simulink model "wind_draiden_proto"  (R2020a)
settings: Solver=ode45  StartTime=0.0  StopTime=20  MaxStep=0.1  RelTol=1e-2  EnableMultiTasking=on
undefined symbols (not defined in the file or in its folder): ln
libraries: simulink x16
settings Model: Creator=Andrey  LastModifiedBy=Tamer
settings SolverCC: AlgebraicLoopSolver=LineSearch
settings DataIOCC: LimitDataPoints=on  SaveFormat=Array  SignalLoggingSaveFormat=ModelDataLogs  ReturnWorkspaceOutputs=off
settings OptimizationCC: InitFltsAndDblsToZero=on  EfficientMapNaN2IntZero=off  LifeSpan=inf
settings DebuggingCC: SaveWithParameterizedLinksMsg=none  UnderspecifiedInitializationDetection=Classic  MergeDetectMultiDrivingBlocksExec=none  SignalResolutionControl=TryResolveAllWithWarning  MaxConsecutiveZCsMsg=none  SolverPrmCheckMsg=warning  MultiTaskDSMMsg=warning  MultiTaskCondExecSysMsg=none  FcnCallInpInsideContextMsg=warning  StateNameClashWarn=warning  SFUnexpectedBacktrackingDiag=warning  SFNoUnconditionalDefaultTransitionDiag=warning  SFExecutionAtInitializationDiag=none  ArithmeticOperatorsInVariantConditions=warning
settings HardwareCC: ProdBitPerPointer=32  ProdBitPerSizeT=32  ProdBitPerPtrDiffT=32  ProdLargestAtomicFloat=None  ProdIntDivRoundTo=Undefined  ProdEndianess=Unspecified  ProdWordSize=32  ProdHWDeviceType=32-bit Generic  TargetBitPerPointer=64  TargetBitPerSizeT=64  TargetBitPerPtrDiffT=64  TargetLongLongMode=on  TargetIntDivRoundTo=Zero  TargetEndianess=LittleEndian  TargetWordSize=64  TargetHWDeviceType=MATLAB Host  ProdEqTarget=off
settings ModelReferenceCC: PropagateSignalLabelsOutOfModel=off
settings SFSimCC: SimUseLocalCustomCode=off  CustomCodeUndefinedFunction=UseInterfaceOnly
settings RTWCC: RTWUseLocalCustomCode=off
settings CodeAppCC: MaxIdLength=128
settings GRTTargetCC: TargetLangStandard=C89/C90 (ANSI)  CombineOutputUpdateFcns=off  GRTInterface=on
settings ConfigComp: CovMetricSettings=dw  CovHtmlReporting=on  CovSaveCumulativeToWorkspaceVar=on  CovSaveSingleToWorkspaceVar=on  CovExternalEMLEnable=off

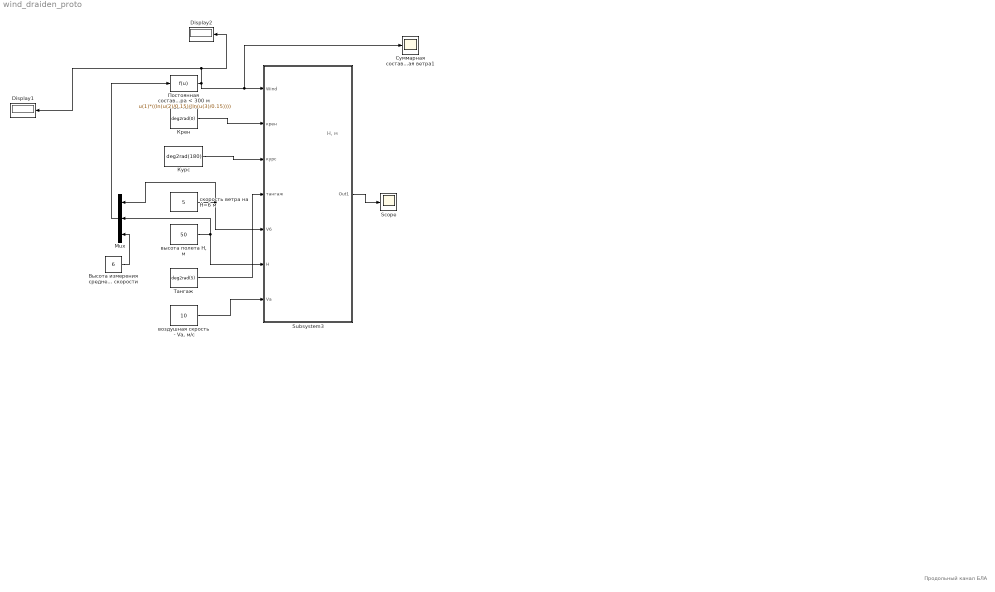
== system wind_draiden_proto ==
  note: Н, м
  note: Продольный канал БЛА
  "    Постоянная составляющая скорости ветра < 300 м" : Fcn  Expr=u(1)*((ln(u(2)/0.15)/(ln(u(3)/0.15))))
  Display1 : Display
  Display2 : Display
  Mux : Mux  Inputs=3
  Scope : Scope
  Subsystem3 : Subsystem
  Высота измерения среднегодовой скорости : Constant  Value=6
  "Крен " : Constant  Value=deg2rad(0)
  Курс : Constant  Value=deg2rad(180)
  Суммарная составляющая ветра1 : Scope
  Тангаж : Constant  Value=deg2rad(5)
  "воздушная скрость  - Vа, м/с" : Constant  Value=10
  "высота полета Н, м " : Constant  Value=50
  "скорость ветра на Н=6 м " : Constant  Value=5
  wires:
  Subsystem3/1(Out1) -> Scope/1
  "Крен "/1 -> Subsystem3/2(крен)
  Курс/1 -> Subsystem3/3(курс)
  "скорость ветра на Н=6 м "/1 -> Subsystem3/5(V6), Mux/1
  "высота полета Н, м "/1 -> Subsystem3/6(H), Mux/2
  Тангаж/1 -> Subsystem3/4("тангаж ")
  "    Постоянная составляющая скорости ветра < 300 м"/1 -> Display2/1, Display1/1, Суммарная составляющая ветра1/1, Subsystem3/1(Wind)
  Высота измерения среднегодовой скорости/1 -> Mux/3
  Mux/1 -> "    Постоянная составляющая скорости ветра < 300 м"/1
  "воздушная скрость  - Vа, м/с"/1 -> Subsystem3/7(Va)

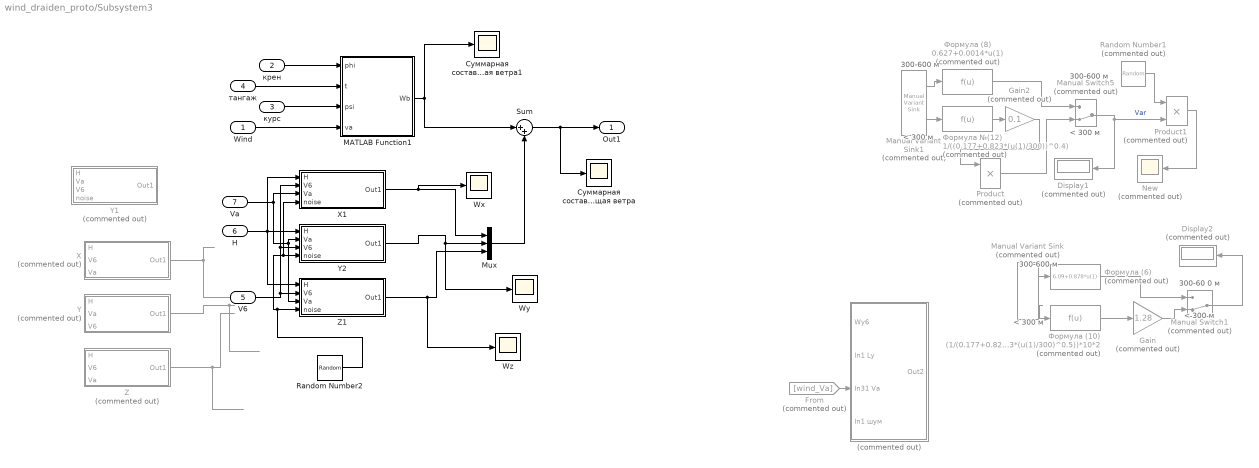
== system wind_draiden_proto/Subsystem3 ==
  note: < 300 м
  note: < 300 м
  note: 300-600 м
  note: < 300 м
  note: 300-60 0 м
  note: 300-600 м
  note: < 300 м
  note: 300-600 м
  Wind : Inport
  крен : Inport  Port=2
  курс : Inport  Port=3
  "тангаж " : Inport  Port=4
  V6 : Inport  Port=5
  H : Inport  Port=6
  Va : Inport  Port=7
  " " : Subsystem  Commented=on
  Display1 : Display  Commented=on
  Display2 : Display  Commented=on
  From : From  Commented=on  GotoTag=wind_Va
  Gain : Gain  Commented=on  Gain=1.28
  Gain2 : Gain  Commented=on  Gain=0.1
  MATLAB Function1 : MATLAB Function  TreatAsAtomicUnit=on
  Manual Variant Sink : simulink/Signal Routing/Manual Variant Sink  Commented=on  NumChoices=2  LabelModeActiveChoice=V_2
  Manual Variant Sink1 : simulink/Signal Routing/Manual Variant Sink  Commented=on  NumChoices=2  LabelModeActiveChoice=V_2
  Manual Switch1 : ManualSwitch  Commented=on  CurrentSetting=0
  Manual Switch5 : ManualSwitch  Commented=on  CurrentSetting=0
  Mux : Mux  Inputs=3
  New : Scope  Commented=on
  Product : Product  Commented=on
  Product1 : Product  Commented=on
  Random Number1 : RandomNumber  Commented=on  SampleTime=0.1
  Random Number2 : RandomNumber  SampleTime=0.1
  Sum : Sum  Inputs=|++
  Wx : Scope
  Wy : Scope
  Wz : Scope
  X : Subsystem  Commented=on  TreatAsAtomicUnit=on
  X1 : Subsystem  TreatAsAtomicUnit=on
  Y : Subsystem  Commented=on  TreatAsAtomicUnit=on
  Y1 : Subsystem  Commented=on  TreatAsAtomicUnit=on
  Y2 : Subsystem  TreatAsAtomicUnit=on
  Z : Subsystem  Commented=on  TreatAsAtomicUnit=on
  Z1 : Subsystem  TreatAsAtomicUnit=on
  Суммарная составляющая ветра : Scope
  Суммарная составляющая ветра1 : Scope
  Формула (10) : Fcn  Commented=on  Expr=(1/(0.177+0.823*(u(1)/300)^0.5))*10*2
  Формула (6) : Fcn  Commented=on  Expr=6.09+0.878*u(1)
  Формула (8) : Fcn  Commented=on  Expr=0.627+0.0014*u(1)
  Формула №(12) : Fcn  Commented=on  Expr=1/((0.177+0.823*(u(1)/300))^0.4)
  Out1 : Outport
  wires:
  Формула (10)/1 -> Gain/1
  Manual Variant Sink/1 -> Формула (6)/1
  Manual Variant Sink/2 -> Формула (10)/1
  крен/1 -> MATLAB Function1/1(phi)
  курс/1 -> MATLAB Function1/3(psi)
  Wind/1 -> MATLAB Function1/4(va)
  Gain2/1 -> Product/1
  Manual Variant Sink1/1 -> Формула (8)/1
  Формула (8)/1 -> Manual Switch5/1
  Формула №(12)/1 -> Gain2/1
  Product/1 -> Manual Switch5/2
  Manual Variant Sink1/2 -> Формула №(12)/1
  Manual Switch5/1 -> Product1/2, Display1/1  "Var"
  Формула (6)/1 -> Manual Switch1/1
  Gain/1 -> Manual Switch1/2
  "тангаж "/1 -> MATLAB Function1/2(t)
  From/1 -> " "/3(In31 Va)
  Manual Switch1/1 -> Display2/1
  Product1/1 -> New/1
  Random Number1/1 -> Product1/1
  MATLAB Function1/1(Wb) -> Sum/1, Суммарная составляющая ветра1/1
  Mux/1 -> Sum/2
  Sum/1 -> Суммарная составляющая ветра/1, Out1/1
  Z/1(Out1) -> ?
  X/1(Out1) -> ?
  Y/1(Out1) -> ?
  Va/1 -> Y2/2(Va), Z1/3(Va), X1/3(Va)
  H/1 -> Y2/1(H), X1/1(H), Z1/1(H)
  V6/1 -> X1/2(V6), Y2/3(V6), Z1/2(V6)
  Z1/1(Out1) -> Wz/1, Mux/3
  X1/1(Out1) -> Mux/1, Wx/1
  Y2/1(Out1) -> Mux/2, Wy/1
  Random Number2/1 -> Y2/4(noise), X1/4(noise), Z1/4(noise)

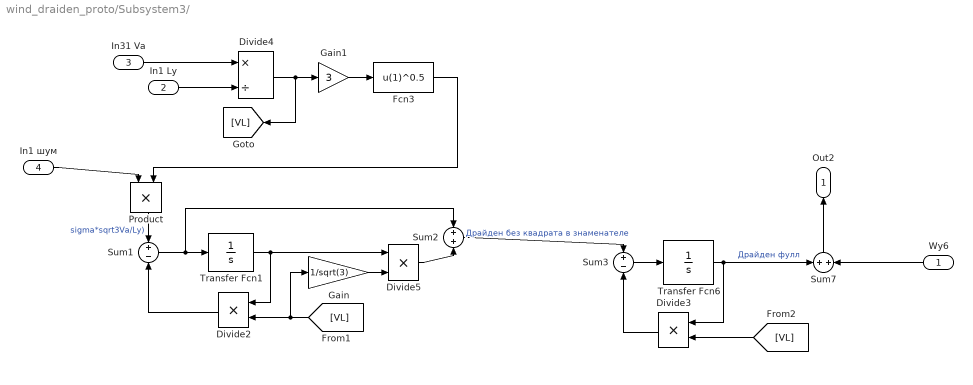
== system wind_draiden_proto/Subsystem3/  ==
  Wy6 : Inport
  In1 Ly : Inport  Port=2
  In31 Va : Inport  Port=3
  "In1 шум " : Inport  Port=4
  Divide2 : Product  Inputs=**
  Divide3 : Product  Inputs=**
  Divide4 : Product  Inputs=*/
  Divide5 : Product  Inputs=**
  Fcn3 : Fcn  Expr=u(1)^0.5
  Gain : Gain  Gain=1/sqrt(3)
  Gain1 : Gain  Gain=3
  Product : Product
  Sum1 : Sum  Inputs=+-
  Sum2 : Sum
  Sum3 : Sum  Inputs=+-
  Sum7 : Sum
  Transfer Fcn1 : TransferFcn  Denominator="[1  0]"
  Transfer Fcn6 : TransferFcn  Denominator="[1  0]"
  Out2 : Outport
  wires:
  Divide4/1 -> [VL], Gain1/1
  Sum1/1 -> Transfer Fcn1/1, Sum2/1
  Sum2/1 -> Sum3/1  "Драйден без квадрата в знаменателе"
  Transfer Fcn1/1 -> Divide2/1, Divide5/1
  Divide2/1 -> Sum1/2
  Gain1/1 -> Fcn3/1
  In31 Va/1 -> Divide4/1
  In1 Ly/1 -> Divide4/2
  [VL] -> Gain/1, Divide2/2
  Gain/1 -> Divide5/2
  Divide5/1 -> Sum2/2
  Transfer Fcn6/1 -> Sum7/1, Divide3/1  "Драйден фулл"
  Divide3/1 -> Sum3/2
  Sum3/1 -> Transfer Fcn6/1
  [VL] -> Divide3/2
  Wy6/1 -> Sum7/2
  Sum7/1 -> Out2/1
  "In1 шум "/1 -> Product/1
  Fcn3/1 -> Product/2
  Product/1 -> Sum1/1  "sigma*sqrt3Va/Ly)"

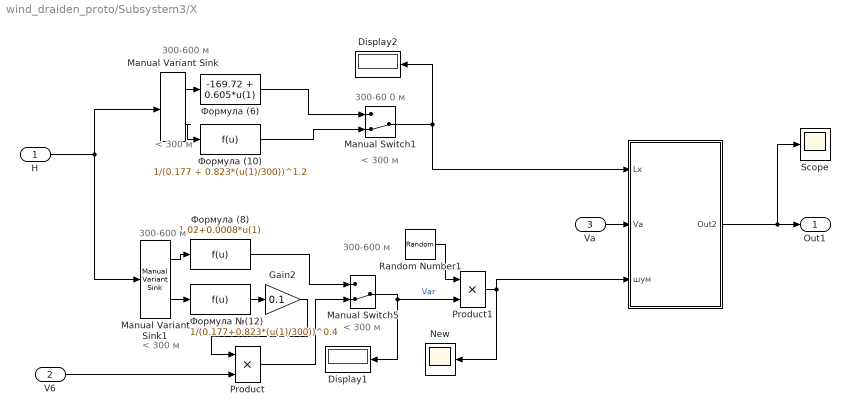
== system wind_draiden_proto/Subsystem3/X ==
  note: < 300 м
  note: 300-600 м
  note: < 300 м
  note: < 300 м
  note: 300-600 м
  note: < 300 м
  note: 300-60 0 м
  note: 300-600 м
  H : Inport
  V6 : Inport  Port=2
  Va : Inport  Port=3
  " " : Subsystem
  Display1 : Display
  Display2 : Display
  Gain2 : Gain  Gain=0.1
  Manual Variant Sink : simulink/Signal Routing/Manual Variant Sink  NumChoices=2  LabelModeActiveChoice=V_2
  Manual Variant Sink1 : simulink/Signal Routing/Manual Variant Sink  NumChoices=2  LabelModeActiveChoice=V_2
  Manual Switch1 : ManualSwitch  CurrentSetting=0
  Manual Switch5 : ManualSwitch  CurrentSetting=0
  New : Scope
  Product : Product
  Product1 : Product
  Random Number1 : RandomNumber  SampleTime=0.1
  Scope : Scope
  Формула (10) : Fcn  Expr=1/(0.177 + 0.823*(u(1)/300))^1.2
  Формула (6) : Fcn  Expr=-169.72 + 0.605*u(1)
  Формула (8) : Fcn  Expr=1.02+0.0008*u(1)
  Формула №(12) : Fcn  Expr=1/(0.177+0.823*(u(1)/300))^0.4
  Out1 : Outport
  wires:
  Random Number1/1 -> Product1/1
  Формула №(12)/1 -> Gain2/1
  Формула (8)/1 -> Manual Switch5/1
  Product1/1 -> New/1, " "/3("шум ")
  Manual Variant Sink/2 -> Формула (10)/1
  Manual Variant Sink1/1 -> Формула (8)/1
  Gain2/1 -> Product/1
  Manual Variant Sink1/2 -> Формула №(12)/1
  Manual Switch5/1 -> Product1/2, Display1/1  "Var"
  " "/1(Out2) -> Scope/1, Out1/1
  Product/1 -> Manual Switch5/2
  Формула (6)/1 -> Manual Switch1/1
  H/1 -> Manual Variant Sink1/1, Manual Variant Sink/1
  V6/1 -> Product/2
  Manual Variant Sink/1 -> Формула (6)/1
  Manual Switch1/1 -> " "/1(Lx), Display2/1
  Формула (10)/1 -> Manual Switch1/2
  Va/1 -> " "/2(Va)

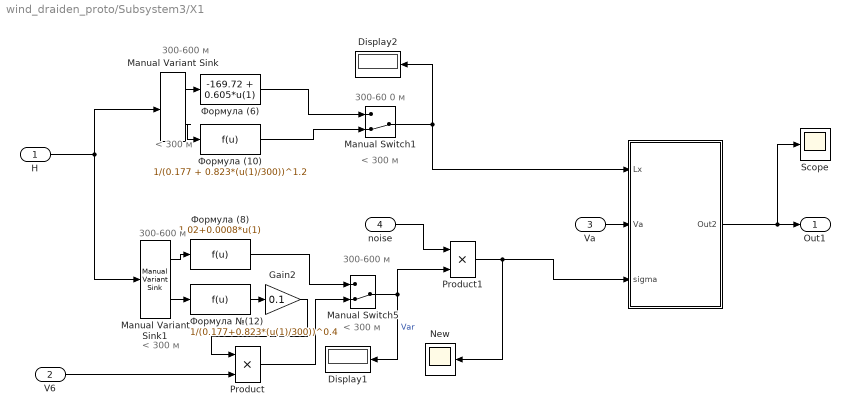
== system wind_draiden_proto/Subsystem3/X1 ==
  note: < 300 м
  note: 300-600 м
  note: < 300 м
  note: < 300 м
  note: 300-600 м
  note: < 300 м
  note: 300-60 0 м
  note: 300-600 м
  H : Inport
  V6 : Inport  Port=2
  Va : Inport  Port=3
  noise : Inport  Port=4
  " " : Subsystem
  Display1 : Display
  Display2 : Display
  Gain2 : Gain  Gain=0.1
  Manual Variant Sink : simulink/Signal Routing/Manual Variant Sink  NumChoices=2  LabelModeActiveChoice=V_2
  Manual Variant Sink1 : simulink/Signal Routing/Manual Variant Sink  NumChoices=2  LabelModeActiveChoice=V_2
  Manual Switch1 : ManualSwitch  CurrentSetting=0
  Manual Switch5 : ManualSwitch  CurrentSetting=0
  New : Scope
  Product : Product
  Product1 : Product
  Scope : Scope
  Формула (10) : Fcn  Expr=1/(0.177 + 0.823*(u(1)/300))^1.2
  Формула (6) : Fcn  Expr=-169.72 + 0.605*u(1)
  Формула (8) : Fcn  Expr=1.02+0.0008*u(1)
  Формула №(12) : Fcn  Expr=1/(0.177+0.823*(u(1)/300))^0.4
  Out1 : Outport
  wires:
  Формула №(12)/1 -> Gain2/1
  Формула (8)/1 -> Manual Switch5/1
  Manual Variant Sink/2 -> Формула (10)/1
  Manual Variant Sink1/1 -> Формула (8)/1
  Gain2/1 -> Product/1
  Manual Variant Sink1/2 -> Формула №(12)/1
  Manual Switch5/1 -> Display1/1, Product1/2  "Var"
  " "/1(Out2) -> Scope/1, Out1/1
  Product/1 -> Manual Switch5/2
  Формула (6)/1 -> Manual Switch1/1
  H/1 -> Manual Variant Sink1/1, Manual Variant Sink/1
  V6/1 -> Product/2
  Manual Variant Sink/1 -> Формула (6)/1
  Manual Switch1/1 -> " "/1(Lx), Display2/1
  Формула (10)/1 -> Manual Switch1/2
  Va/1 -> " "/2(Va)
  Product1/1 -> New/1, " "/3("sigma ")
  noise/1 -> Product1/1

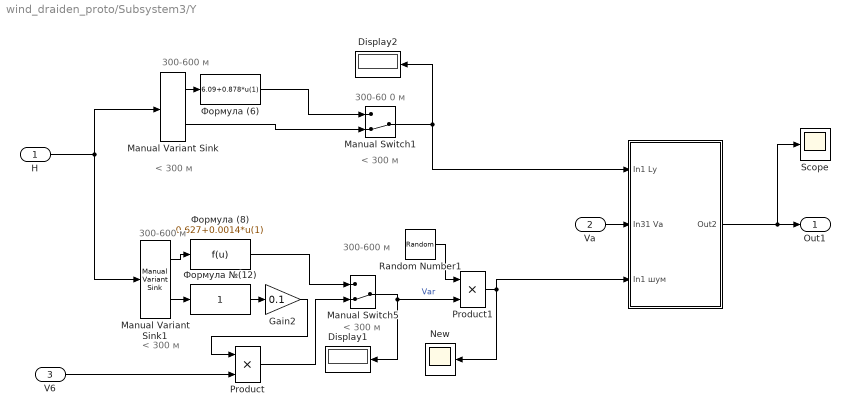
== system wind_draiden_proto/Subsystem3/Y ==
  note: < 300 м
  note: 300-600 м
  note: < 300 м
  note: < 300 м
  note: 300-600 м
  note: < 300 м
  note: 300-60 0 м
  note: 300-600 м
  H : Inport
  Va : Inport  Port=2
  V6 : Inport  Port=3
  " " : Subsystem
  Display1 : Display
  Display2 : Display
  Gain2 : Gain  Gain=0.1
  Manual Variant Sink : simulink/Signal Routing/Manual Variant Sink  NumChoices=2  LabelModeActiveChoice=V_2
  Manual Variant Sink1 : simulink/Signal Routing/Manual Variant Sink  NumChoices=2  LabelModeActiveChoice=V_2
  Manual Switch1 : ManualSwitch  CurrentSetting=0
  Manual Switch5 : ManualSwitch  CurrentSetting=0
  New : Scope
  Product : Product
  Product1 : Product
  Random Number1 : RandomNumber  SampleTime=0.1
  Scope : Scope
  Формула (6) : Fcn  Expr=6.09+0.878*u(1)
  Формула (8) : Fcn  Expr=0.627+0.0014*u(1)
  Формула №(12) : Fcn  Expr=1
  Out1 : Outport
  wires:
  Random Number1/1 -> Product1/1
  Формула №(12)/1 -> Gain2/1
  Формула (8)/1 -> Manual Switch5/1
  Product1/1 -> New/1, " "/3("In1 шум ")
  Manual Variant Sink1/1 -> Формула (8)/1
  Gain2/1 -> Product/1
  Manual Variant Sink1/2 -> Формула №(12)/1
  Manual Switch5/1 -> Product1/2, Display1/1  "Var"
  " "/1(Out2) -> Scope/1, Out1/1
  Product/1 -> Manual Switch5/2
  Формула (6)/1 -> Manual Switch1/1
  H/1 -> Manual Variant Sink1/1, Manual Variant Sink/1
  V6/1 -> Product/2
  Manual Variant Sink/1 -> Формула (6)/1
  Manual Switch1/1 -> " "/1(In1 Ly), Display2/1
  Manual Variant Sink/2 -> Manual Switch1/2
  Va/1 -> " "/2(In31 Va)

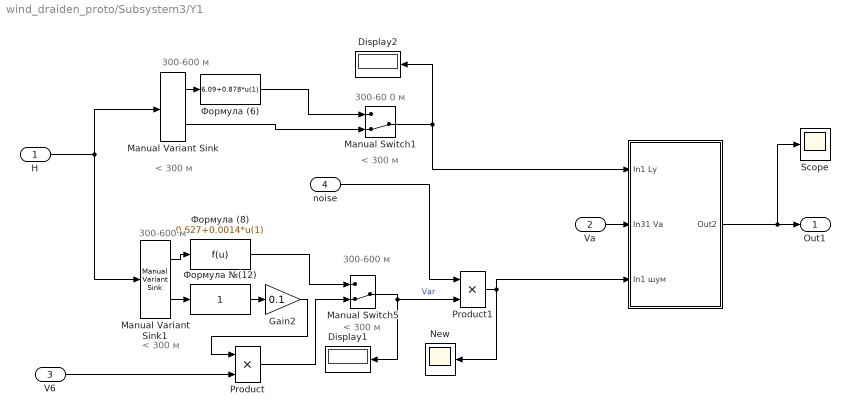
== system wind_draiden_proto/Subsystem3/Y1 ==
  note: < 300 м
  note: 300-600 м
  note: < 300 м
  note: < 300 м
  note: 300-600 м
  note: < 300 м
  note: 300-60 0 м
  note: 300-600 м
  H : Inport
  Va : Inport  Port=2
  V6 : Inport  Port=3
  noise : Inport  Port=4
  " " : Subsystem
  Display1 : Display
  Display2 : Display
  Gain2 : Gain  Gain=0.1
  Manual Variant Sink : simulink/Signal Routing/Manual Variant Sink  NumChoices=2  LabelModeActiveChoice=V_2
  Manual Variant Sink1 : simulink/Signal Routing/Manual Variant Sink  NumChoices=2  LabelModeActiveChoice=V_2
  Manual Switch1 : ManualSwitch  CurrentSetting=0
  Manual Switch5 : ManualSwitch  CurrentSetting=0
  New : Scope
  Product : Product
  Product1 : Product
  Scope : Scope
  Формула (6) : Fcn  Expr=6.09+0.878*u(1)
  Формула (8) : Fcn  Expr=0.627+0.0014*u(1)
  Формула №(12) : Fcn  Expr=1
  Out1 : Outport
  wires:
  noise/1 -> Product1/1
  Формула №(12)/1 -> Gain2/1
  Формула (8)/1 -> Manual Switch5/1
  Product1/1 -> " "/3("In1 шум "), New/1
  Manual Variant Sink1/1 -> Формула (8)/1
  Gain2/1 -> Product/1
  Manual Variant Sink1/2 -> Формула №(12)/1
  Manual Switch5/1 -> Product1/2, Display1/1  "Var"
  " "/1(Out2) -> Scope/1, Out1/1
  Product/1 -> Manual Switch5/2
  Формула (6)/1 -> Manual Switch1/1
  H/1 -> Manual Variant Sink1/1, Manual Variant Sink/1
  V6/1 -> Product/2
  Manual Variant Sink/1 -> Формула (6)/1
  Manual Switch1/1 -> " "/1(In1 Ly), Display2/1
  Manual Variant Sink/2 -> Manual Switch1/2
  Va/1 -> " "/2(In31 Va)

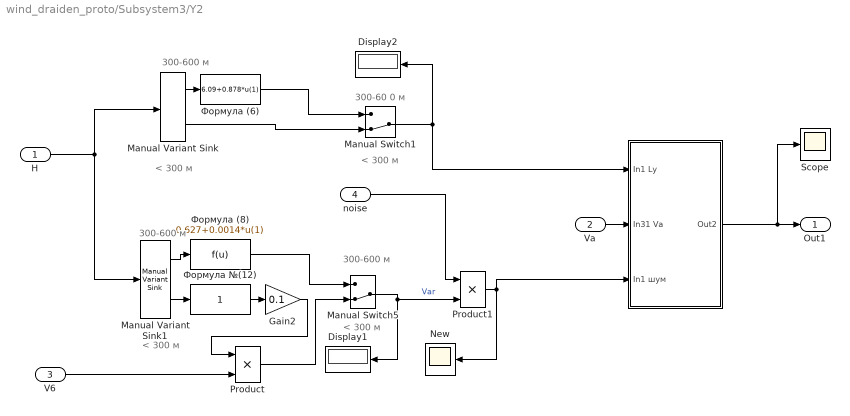
== system wind_draiden_proto/Subsystem3/Y2 ==
  note: < 300 м
  note: 300-600 м
  note: < 300 м
  note: < 300 м
  note: 300-600 м
  note: < 300 м
  note: 300-60 0 м
  note: 300-600 м
  H : Inport
  Va : Inport  Port=2
  V6 : Inport  Port=3
  noise : Inport  Port=4
  " " : Subsystem
  Display1 : Display
  Display2 : Display
  Gain2 : Gain  Gain=0.1
  Manual Variant Sink : simulink/Signal Routing/Manual Variant Sink  NumChoices=2  LabelModeActiveChoice=V_2
  Manual Variant Sink1 : simulink/Signal Routing/Manual Variant Sink  NumChoices=2  LabelModeActiveChoice=V_2
  Manual Switch1 : ManualSwitch  CurrentSetting=0
  Manual Switch5 : ManualSwitch  CurrentSetting=0
  New : Scope
  Product : Product
  Product1 : Product
  Scope : Scope
  Формула (6) : Fcn  Expr=6.09+0.878*u(1)
  Формула (8) : Fcn  Expr=0.627+0.0014*u(1)
  Формула №(12) : Fcn  Expr=1
  Out1 : Outport
  wires:
  noise/1 -> Product1/1
  Формула №(12)/1 -> Gain2/1
  Формула (8)/1 -> Manual Switch5/1
  Product1/1 -> New/1, " "/3("In1 шум ")
  Manual Variant Sink1/1 -> Формула (8)/1
  Gain2/1 -> Product/1
  Manual Variant Sink1/2 -> Формула №(12)/1
  Manual Switch5/1 -> Product1/2, Display1/1  "Var"
  " "/1(Out2) -> Scope/1, Out1/1
  Product/1 -> Manual Switch5/2
  Формула (6)/1 -> Manual Switch1/1
  H/1 -> Manual Variant Sink1/1, Manual Variant Sink/1
  V6/1 -> Product/2
  Manual Variant Sink/1 -> Формула (6)/1
  Manual Switch1/1 -> " "/1(In1 Ly), Display2/1
  Manual Variant Sink/2 -> Manual Switch1/2
  Va/1 -> " "/2(In31 Va)

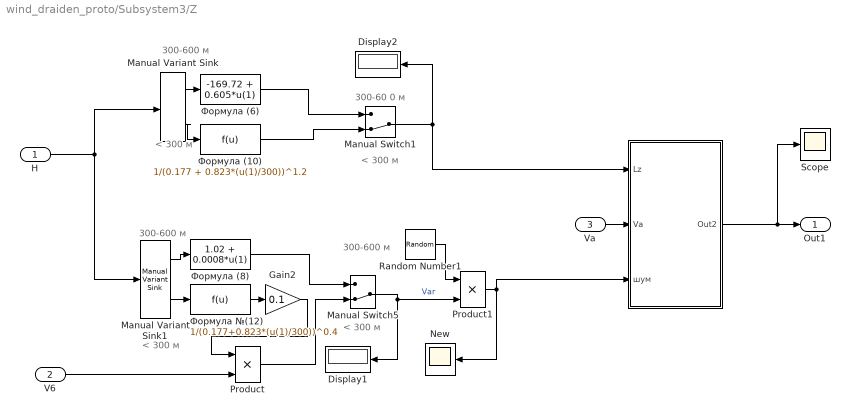
== system wind_draiden_proto/Subsystem3/Z ==
  note: < 300 м
  note: 300-600 м
  note: < 300 м
  note: < 300 м
  note: 300-600 м
  note: < 300 м
  note: 300-60 0 м
  note: 300-600 м
  H : Inport
  V6 : Inport  Port=2
  Va : Inport  Port=3
  " " : Subsystem
  Display1 : Display
  Display2 : Display
  Gain2 : Gain  Gain=0.1
  Manual Variant Sink : simulink/Signal Routing/Manual Variant Sink  NumChoices=2  LabelModeActiveChoice=V_2
  Manual Variant Sink1 : simulink/Signal Routing/Manual Variant Sink  NumChoices=2  LabelModeActiveChoice=V_2
  Manual Switch1 : ManualSwitch  CurrentSetting=0
  Manual Switch5 : ManualSwitch  CurrentSetting=0
  New : Scope
  Product : Product
  Product1 : Product
  Random Number1 : RandomNumber  SampleTime=0.1
  Scope : Scope
  Формула (10) : Fcn  Expr=1/(0.177 + 0.823*(u(1)/300))^1.2
  Формула (6) : Fcn  Expr=-169.72 + 0.605*u(1)
  Формула (8) : Fcn  Expr=1.02 + 0.0008*u(1)
  Формула №(12) : Fcn  Expr=1/(0.177+0.823*(u(1)/300))^0.4
  Out1 : Outport
  wires:
  Random Number1/1 -> Product1/1
  Формула №(12)/1 -> Gain2/1
  Формула (8)/1 -> Manual Switch5/1
  Product1/1 -> New/1, " "/3("шум ")
  Manual Variant Sink/2 -> Формула (10)/1
  Manual Variant Sink1/1 -> Формула (8)/1
  Gain2/1 -> Product/1
  Manual Variant Sink1/2 -> Формула №(12)/1
  Manual Switch5/1 -> Product1/2, Display1/1  "Var"
  " "/1(Out2) -> Scope/1, Out1/1
  Product/1 -> Manual Switch5/2
  Формула (6)/1 -> Manual Switch1/1
  H/1 -> Manual Variant Sink1/1, Manual Variant Sink/1
  V6/1 -> Product/2
  Manual Variant Sink/1 -> Формула (6)/1
  Manual Switch1/1 -> " "/1(Lz), Display2/1
  Формула (10)/1 -> Manual Switch1/2
  Va/1 -> " "/2(Va)

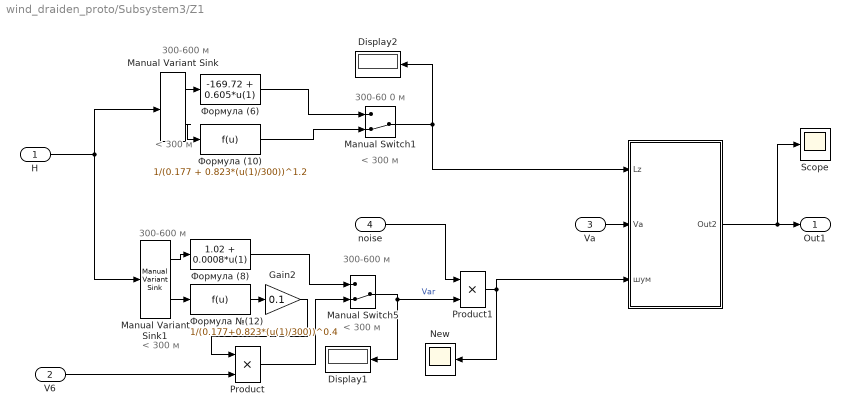
== system wind_draiden_proto/Subsystem3/Z1 ==
  note: < 300 м
  note: 300-600 м
  note: < 300 м
  note: < 300 м
  note: 300-600 м
  note: < 300 м
  note: 300-60 0 м
  note: 300-600 м
  H : Inport
  V6 : Inport  Port=2
  Va : Inport  Port=3
  noise : Inport  Port=4
  " " : Subsystem
  Display1 : Display
  Display2 : Display
  Gain2 : Gain  Gain=0.1
  Manual Variant Sink : simulink/Signal Routing/Manual Variant Sink  NumChoices=2  LabelModeActiveChoice=V_2
  Manual Variant Sink1 : simulink/Signal Routing/Manual Variant Sink  NumChoices=2  LabelModeActiveChoice=V_2
  Manual Switch1 : ManualSwitch  CurrentSetting=0
  Manual Switch5 : ManualSwitch  CurrentSetting=0
  New : Scope
  Product : Product
  Product1 : Product
  Scope : Scope
  Формула (10) : Fcn  Expr=1/(0.177 + 0.823*(u(1)/300))^1.2
  Формула (6) : Fcn  Expr=-169.72 + 0.605*u(1)
  Формула (8) : Fcn  Expr=1.02 + 0.0008*u(1)
  Формула №(12) : Fcn  Expr=1/(0.177+0.823*(u(1)/300))^0.4
  Out1 : Outport
  wires:
  noise/1 -> Product1/1
  Формула №(12)/1 -> Gain2/1
  Формула (8)/1 -> Manual Switch5/1
  Product1/1 -> New/1, " "/3("шум ")
  Manual Variant Sink/2 -> Формула (10)/1
  Manual Variant Sink1/1 -> Формула (8)/1
  Gain2/1 -> Product/1
  Manual Variant Sink1/2 -> Формула №(12)/1
  Manual Switch5/1 -> Product1/2, Display1/1  "Var"
  " "/1(Out2) -> Scope/1, Out1/1
  Product/1 -> Manual Switch5/2
  Формула (6)/1 -> Manual Switch1/1
  H/1 -> Manual Variant Sink1/1, Manual Variant Sink/1
  V6/1 -> Product/2
  Manual Variant Sink/1 -> Формула (6)/1
  Manual Switch1/1 -> " "/1(Lz), Display2/1
  Формула (10)/1 -> Manual Switch1/2
  Va/1 -> " "/2(Va)

== system wind_draiden_proto/Subsystem3/X/  ==
  Lx : Inport
  Va : Inport  Port=2
  "шум " : Inport  Port=3
  Divide3 : Product  Inputs=**
  Divide4 : Product  Inputs=*/
  Fcn3 : Fcn  Expr=u(1)^0.5
  Gain1 : Gain  Gain=2
  Product : Product
  Sum3 : Sum  Inputs=+-
  Transfer Fcn6 : TransferFcn  Denominator="[1  0]"
  Out2 : Outport
  wires:
  Divide4/1 -> [VL], Gain1/1
  Gain1/1 -> Fcn3/1
  Va/1 -> Divide4/1
  Lx/1 -> Divide4/2
  Transfer Fcn6/1 -> Out2/1, Divide3/1  "Драйден фулл"
  Divide3/1 -> Sum3/2
  Sum3/1 -> Transfer Fcn6/1
  [VL] -> Divide3/2
  "шум "/1 -> Product/1
  Fcn3/1 -> Product/2
  Product/1 -> Sum3/1  "sigma*Va/Lx)"

== system wind_draiden_proto/Subsystem3/X1/  ==
  Lx : Inport
  Va : Inport  Port=2
  "sigma " : Inport  Port=3
  Divide3 : Product  Inputs=**
  Divide4 : Product  Inputs=*/
  Fcn3 : Fcn  Expr=u(1)^0.5
  Gain1 : Gain  Gain=2
  Product : Product
  Sum3 : Sum  Inputs=+-
  Transfer Fcn6 : TransferFcn  Denominator="[1  0]"
  Out2 : Outport
  wires:
  Divide4/1 -> [VL], Gain1/1
  Gain1/1 -> Fcn3/1
  Va/1 -> Divide4/1
  Lx/1 -> Divide4/2
  Transfer Fcn6/1 -> Out2/1, Divide3/1  "Драйден фулл"
  Divide3/1 -> Sum3/2
  Sum3/1 -> Transfer Fcn6/1
  [VL] -> Divide3/2
  Product/1 -> Sum3/1  "sigma*Va/Lx)"
  "sigma "/1 -> Product/1
  Fcn3/1 -> Product/2

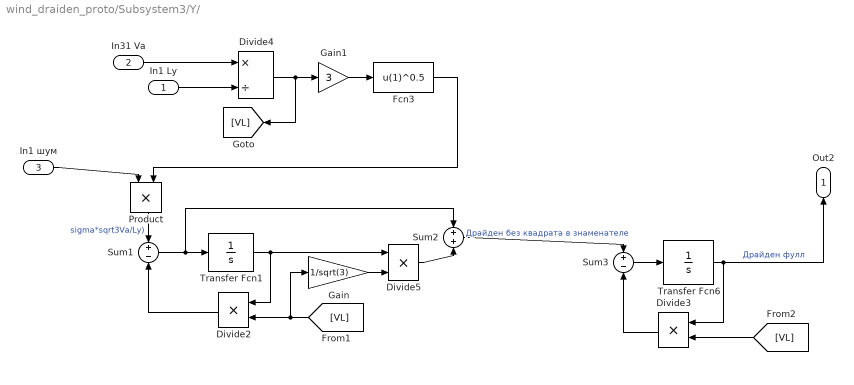
== system wind_draiden_proto/Subsystem3/Y/  ==
  In1 Ly : Inport
  In31 Va : Inport  Port=2
  "In1 шум " : Inport  Port=3
  Divide2 : Product  Inputs=**
  Divide3 : Product  Inputs=**
  Divide4 : Product  Inputs=*/
  Divide5 : Product  Inputs=**
  Fcn3 : Fcn  Expr=u(1)^0.5
  Gain : Gain  Gain=1/sqrt(3)
  Gain1 : Gain  Gain=3
  Product : Product
  Sum1 : Sum  Inputs=+-
  Sum2 : Sum
  Sum3 : Sum  Inputs=+-
  Transfer Fcn1 : TransferFcn  Denominator="[1  0]"
  Transfer Fcn6 : TransferFcn  Denominator="[1  0]"
  Out2 : Outport
  wires:
  Divide4/1 -> [VL], Gain1/1
  Sum1/1 -> Transfer Fcn1/1, Sum2/1
  Sum2/1 -> Sum3/1  "Драйден без квадрата в знаменателе"
  Transfer Fcn1/1 -> Divide2/1, Divide5/1
  Divide2/1 -> Sum1/2
  Gain1/1 -> Fcn3/1
  In31 Va/1 -> Divide4/1
  In1 Ly/1 -> Divide4/2
  [VL] -> Gain/1, Divide2/2
  Gain/1 -> Divide5/2
  Divide5/1 -> Sum2/2
  Transfer Fcn6/1 -> Out2/1, Divide3/1  "Драйден фулл"
  Divide3/1 -> Sum3/2
  Sum3/1 -> Transfer Fcn6/1
  [VL] -> Divide3/2
  "In1 шум "/1 -> Product/1
  Fcn3/1 -> Product/2
  Product/1 -> Sum1/1  "sigma*sqrt3Va/Ly)"

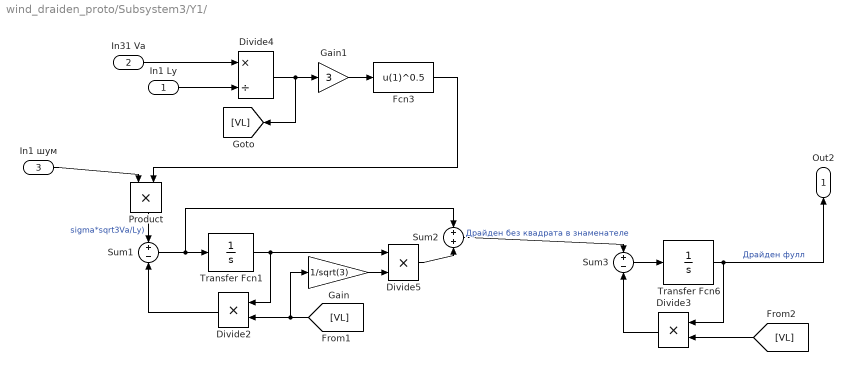
== system wind_draiden_proto/Subsystem3/Y1/  ==
  In1 Ly : Inport
  In31 Va : Inport  Port=2
  "In1 шум " : Inport  Port=3
  Divide2 : Product  Inputs=**
  Divide3 : Product  Inputs=**
  Divide4 : Product  Inputs=*/
  Divide5 : Product  Inputs=**
  Fcn3 : Fcn  Expr=u(1)^0.5
  Gain : Gain  Gain=1/sqrt(3)
  Gain1 : Gain  Gain=3
  Product : Product
  Sum1 : Sum  Inputs=+-
  Sum2 : Sum
  Sum3 : Sum  Inputs=+-
  Transfer Fcn1 : TransferFcn  Denominator="[1  0]"
  Transfer Fcn6 : TransferFcn  Denominator="[1  0]"
  Out2 : Outport
  wires:
  Divide4/1 -> [VL], Gain1/1
  Sum1/1 -> Transfer Fcn1/1, Sum2/1
  Sum2/1 -> Sum3/1  "Драйден без квадрата в знаменателе"
  Transfer Fcn1/1 -> Divide2/1, Divide5/1
  Divide2/1 -> Sum1/2
  Gain1/1 -> Fcn3/1
  In31 Va/1 -> Divide4/1
  In1 Ly/1 -> Divide4/2
  [VL] -> Gain/1, Divide2/2
  Gain/1 -> Divide5/2
  Divide5/1 -> Sum2/2
  Transfer Fcn6/1 -> Out2/1, Divide3/1  "Драйден фулл"
  Divide3/1 -> Sum3/2
  Sum3/1 -> Transfer Fcn6/1
  [VL] -> Divide3/2
  "In1 шум "/1 -> Product/1
  Fcn3/1 -> Product/2
  Product/1 -> Sum1/1  "sigma*sqrt3Va/Ly)"

== system wind_draiden_proto/Subsystem3/Y2/  ==
  In1 Ly : Inport
  In31 Va : Inport  Port=2
  "In1 шум " : Inport  Port=3
  Divide2 : Product  Inputs=**
  Divide3 : Product  Inputs=**
  Divide4 : Product  Inputs=*/
  Divide5 : Product  Inputs=**
  Fcn3 : Fcn  Expr=u(1)^0.5
  Gain : Gain  Gain=1/sqrt(3)
  Gain1 : Gain  Gain=3
  Product : Product
  Sum1 : Sum  Inputs=+-
  Sum2 : Sum
  Sum3 : Sum  Inputs=+-
  Transfer Fcn1 : TransferFcn  Denominator="[1  0]"
  Transfer Fcn6 : TransferFcn  Denominator="[1  0]"
  Out2 : Outport
  wires:
  Divide4/1 -> [VL], Gain1/1
  Sum1/1 -> Transfer Fcn1/1, Sum2/1
  Sum2/1 -> Sum3/1  "Драйден без квадрата в знаменателе"
  Transfer Fcn1/1 -> Divide2/1, Divide5/1
  Divide2/1 -> Sum1/2
  Gain1/1 -> Fcn3/1
  In31 Va/1 -> Divide4/1
  In1 Ly/1 -> Divide4/2
  [VL] -> Gain/1, Divide2/2
  Gain/1 -> Divide5/2
  Divide5/1 -> Sum2/2
  Transfer Fcn6/1 -> Out2/1, Divide3/1  "Драйден фулл"
  Divide3/1 -> Sum3/2
  Sum3/1 -> Transfer Fcn6/1
  [VL] -> Divide3/2
  "In1 шум "/1 -> Product/1
  Fcn3/1 -> Product/2
  Product/1 -> Sum1/1  "sigma*sqrt3Va/Ly)"

== system wind_draiden_proto/Subsystem3/Z/  ==
  Lz : Inport
  Va : Inport  Port=2
  "шум " : Inport  Port=3
  Divide2 : Product  Inputs=**
  Divide3 : Product  Inputs=**
  Divide4 : Product  Inputs=*/
  Divide5 : Product  Inputs=**
  Fcn3 : Fcn  Expr=u(1)^0.5
  Gain : Gain  Gain=1/sqrt(3)
  Gain1 : Gain  Gain=3
  Product : Product
  Sum1 : Sum  Inputs=+-
  Sum2 : Sum
  Sum3 : Sum  Inputs=+-
  Transfer Fcn1 : TransferFcn  Denominator="[1  0]"
  Transfer Fcn6 : TransferFcn  Denominator="[1  0]"
  Out2 : Outport
  wires:
  Divide4/1 -> [VL], Gain1/1
  Sum1/1 -> Transfer Fcn1/1, Sum2/1
  Sum2/1 -> Sum3/1  "Драйден без квадрата в знаменателе"
  Transfer Fcn1/1 -> Divide2/1, Divide5/1
  Divide2/1 -> Sum1/2
  Gain1/1 -> Fcn3/1
  Va/1 -> Divide4/1
  Lz/1 -> Divide4/2
  [VL] -> Gain/1, Divide2/2
  Gain/1 -> Divide5/2
  Divide5/1 -> Sum2/2
  Transfer Fcn6/1 -> Out2/1, Divide3/1  "Драйден фулл"
  Divide3/1 -> Sum3/2
  Sum3/1 -> Transfer Fcn6/1
  [VL] -> Divide3/2
  "шум "/1 -> Product/1
  Fcn3/1 -> Product/2
  Product/1 -> Sum1/1  "sigma*sqrt3Va/Lz)"

== system wind_draiden_proto/Subsystem3/Z1/  ==
  Lz : Inport
  Va : Inport  Port=2
  "шум " : Inport  Port=3
  Divide2 : Product  Inputs=**
  Divide3 : Product  Inputs=**
  Divide4 : Product  Inputs=*/
  Divide5 : Product  Inputs=**
  Fcn3 : Fcn  Expr=u(1)^0.5
  Gain : Gain  Gain=1/sqrt(3)
  Gain1 : Gain  Gain=3
  Product : Product
  Sum1 : Sum  Inputs=+-
  Sum2 : Sum
  Sum3 : Sum  Inputs=+-
  Transfer Fcn1 : TransferFcn  Denominator="[1  0]"
  Transfer Fcn6 : TransferFcn  Denominator="[1  0]"
  Out2 : Outport
  wires:
  Divide4/1 -> [VL], Gain1/1
  Sum1/1 -> Transfer Fcn1/1, Sum2/1
  Sum2/1 -> Sum3/1  "Драйден без квадрата в знаменателе"
  Transfer Fcn1/1 -> Divide2/1, Divide5/1
  Divide2/1 -> Sum1/2
  Gain1/1 -> Fcn3/1
  Va/1 -> Divide4/1
  Lz/1 -> Divide4/2
  [VL] -> Gain/1, Divide2/2
  Gain/1 -> Divide5/2
  Divide5/1 -> Sum2/2
  Transfer Fcn6/1 -> Out2/1, Divide3/1  "Драйден фулл"
  Divide3/1 -> Sum3/2
  Sum3/1 -> Transfer Fcn6/1
  [VL] -> Divide3/2
  "шум "/1 -> Product/1
  Fcn3/1 -> Product/2
  Product/1 -> Sum1/1  "sigma*sqrt3Va/Lz)"

== matlab function wind_draiden_proto/Subsystem3/MATLAB Function1 ==
  data: phi input; Wb output; t input; psi input; va input
function Wb = rotate_g_b(phi, t, psi, va)
R = getRotationMatrix([phi t psi]);
vay=0; vaz=0;
Va = [va; vay; vaz];
Wb = R*Va;

function R = getRotationMatrix(angles)
    phi = 1; t = 2; psi = 3; %indices
    s = sin(angles);
    c = cos(angles);
    R = [
        c(t)*c(psi) s(t)    -c(t)*s(psi);
        -c(phi)*s(t)*c(psi)+s(phi)*s(psi) c(phi)*c(t) c(phi)*s(t)*s(psi)+s(phi)*c(psi);
        s(phi)*s(t)*c(psi)+c(phi)*s(psi)  -s(phi)*c(t)    -s(psi)*s(t)*s(phi)+c(psi)*c(phi);
    ];
